simulink model "TP2"  (R2023b)
settings: Solver=VariableStepAuto  StartTime=0.0  StopTime=2  RelTol=1e-3
settings Model: Creator=ousso  LastModifiedBy=ousso

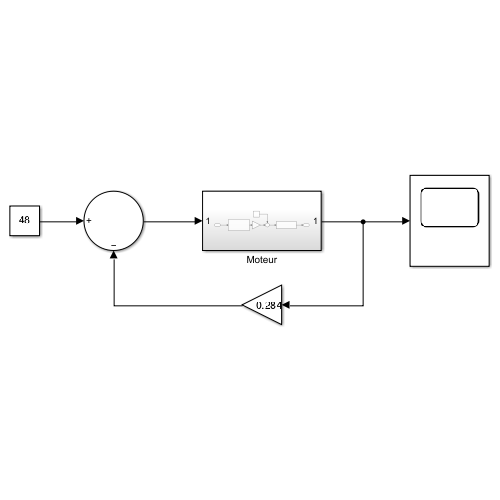
[thumbnail: Simulink's stored preview of the top-level diagram]
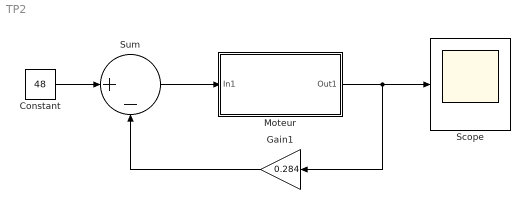
== system TP2 ==
  Constant : Constant  Value=48
  Gain1 : Gain  Gain=0.284
  Moteur : Subsystem
  Scope : Scope
  Sum : Sum  Inputs=|+-
  wires:
  Sum/1 -> Moteur/1(In1)
  Gain1/1 -> Sum/2
  Constant/1 -> Sum/1
  Moteur/1(Out1) -> Gain1/1, Scope/1

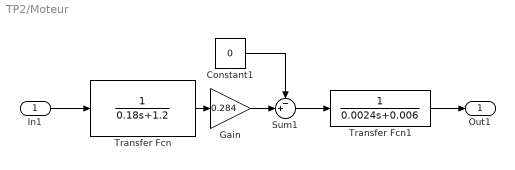
== system TP2/Moteur ==
  In1 : Inport
  Constant1 : Constant  Value=0
  Gain : Gain  Gain=0.284
  Sum1 : Sum  Inputs=-+|
  Transfer Fcn : TransferFcn  Denominator=[0.18 1.2]
  Transfer Fcn1 : TransferFcn  Denominator=[0.0024 0.006]
  Out1 : Outport
  wires:
  Sum1/1 -> Transfer Fcn1/1
  Constant1/1 -> Sum1/1
  Gain/1 -> Sum1/2
  Transfer Fcn/1 -> Gain/1
  In1/1 -> Transfer Fcn/1
  Transfer Fcn1/1 -> Out1/1
